simulink model "fig2_43_simulink"  (R2021b)
settings: Solver=ode45  StartTime=0.0  StopTime=20  RelTol=1e-3  EnableMultiTasking=on
settings Model: Creator=One Informatic  LastModifiedBy=One Informatic
settings DataIOCC: LimitDataPoints=on  SaveFormat=Array  SignalLoggingSaveFormat=ModelDataLogs  ReturnWorkspaceOutputs=off  SignalLoggingName=sigsOut
settings DebuggingCC: SaveWithParameterizedLinksMsg=none  UnderspecifiedInitializationDetection=Classic  MergeDetectMultiDrivingBlocksExec=none  SignalResolutionControl=TryResolveAllWithWarning  MultiTaskDSMMsg=warning  MultiTaskCondExecSysMsg=none
settings HardwareCC: ProdBitPerPointer=32  ProdBitPerSizeT=32  ProdBitPerPtrDiffT=32  ProdLargestAtomicFloat=None  ProdIntDivRoundTo=Undefined  ProdEndianess=Unspecified  ProdWordSize=32  ProdHWDeviceType=32-bit Generic  TargetUnknown=on
settings ModelReferenceCC: PropagateSignalLabelsOutOfModel=off
settings GRTTargetCC: CombineOutputUpdateFcns=off  GRTInterface=on
settings ConfigComp: CovMetricSettings=dw  CovSaveCumulativeToWorkspaceVar=on  CovSaveSingleToWorkspaceVar=on

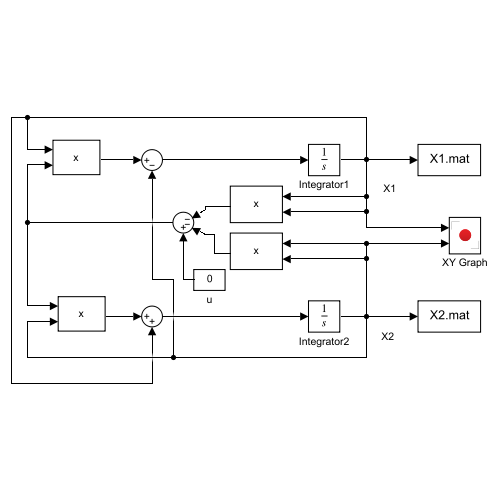
[thumbnail: Simulink's stored preview of the top-level diagram]
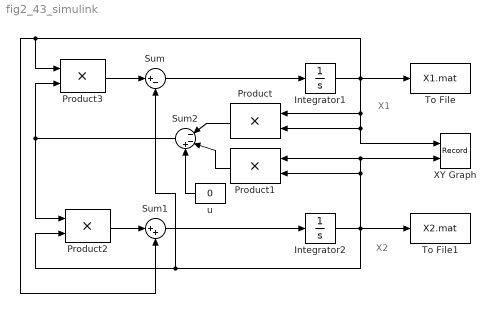
== system fig2_43_simulink ==
  note: X1
  note: X2
  Integrator1 : Integrator  InitialCondition=-2.2
  Integrator2 : Integrator  InitialCondition=1
  Product{,1..3} (4 alike) : Product  SaturateOnIntegerOverflow=on  OutDataTypeStr=Inherit: Same as first input
  Sum : Sum  Inputs=|+-  SaturateOnIntegerOverflow=on
  Sum1 : Sum  Inputs=|++  SaturateOnIntegerOverflow=on
  Sum2 : Sum  Inputs=|--+  SaturateOnIntegerOverflow=on
  To File : ToFile  Filename=X1.mat  MatrixName=X1  SampleTime=0.001
  To File1 : ToFile  Filename=X2.mat  MatrixName=X2  SampleTime=0.001
  XY Graph : Record  FileSettingsInternal="{\"entries\":[{\"content\":{\"excelSettings\":{\"content\":{},\"type\":\"Streamout.ExcelSettings\"}},\"type\":\"Streamout.FileSettingStorage\",\"uuid\":\"dae918f3-7d2f-479d-a086-fab08fd9a2cf\"}],\"packageUris\":[\"http://schema.mathworks.com/mf0/streamout_blocks/R2020a\"],\"version\":\"1.0\"}"  Layout=[1 1]  SignalsInternal="{\"entries\":[{\"content\":{\"signals\":[{\"content\":{\"blockPath\":[\"fig2_43_simulink/XY Graph\"],\"channel\":[],\"dimensions\":[1],\"domain\":\"fig2_43_simulink/XY Graph\",\"lineColor\":\"#ff6929\",\"plots\":[],\"port\":1,\"sid\":[],\"signalID\":36,\"signalName\":\"Integrator1\"},\"type\":\"RecordBlkView.Signal\",\"uuid\":\"3c4a668d-cda4-4d93-b850-ba371b439610\"},{\"content\":{\"blockPath\":[\"fig2_43_simulink/XY Graph\"],\"channel\":[],\"dimensions\":[1],\"domain\":\"fig2_43_simulink/XY Graph\",\"lineColor\":\"#b746ff\",\"plots\":[],\"port\":2,\"sid\":[],\"signalID\":39,\"signalName\":\"Integrator2\"},\"type\":\"RecordBlkView.Signal\",\"uuid\":\"86a1b898-4a79-4262-a09b-3582a0c65380\"}]},\"type\":\"RecordBlkView.InputSignals\",\"uuid\":\"0a0ebd46-1cb9-4a60-9d58-64c83a707fb8\"}],\"packageUris\":[\"http://schema.mathworks.com/mf0/streamout_blocks/R2020a\"],\"version\":\"1.0\"}"  VisualizationBindings="{\"xyplotplugin\":{\"info\":[{\"series\":[],\"subplotID\":1}]}}"  CompatibilityTag=XY  st=0.02
  u : Constant  Value=0
  wires:
  Product/1 -> Sum2/1
  Product1/1 -> Sum2/2
  u/1 -> Sum2/3
  Integrator1/1 -> To File/1, Product/1, Product/2, XY Graph/1, Product3/1, Sum1/2
  Sum2/1 -> Product3/2, Product2/1
  Sum/1 -> Integrator1/1
  Product3/1 -> Sum/1
  Sum1/1 -> Integrator2/1
  Product2/1 -> Sum1/1
  Integrator2/1 -> To File1/1, Product1/1, XY Graph/2, Product1/2, Product2/2, Sum/2
